simulink model "Figure8"  (R2021b)
settings: Solver=VariableStepAuto  StartTime=0.0  StopTime=10.0  RelTol=1e-3
undefined symbols (not defined in the file or in its folder): get, gray, res
libraries: myLib_CustomBoolean x15, dspobslib x1
settings Model: Creator=matt  LastModifiedBy=matt

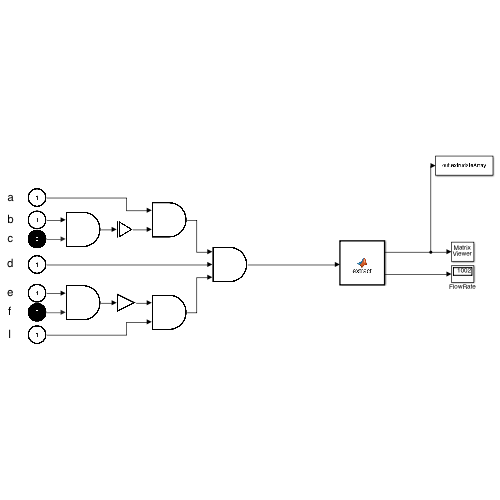
[thumbnail: Simulink's stored preview of the top-level diagram]
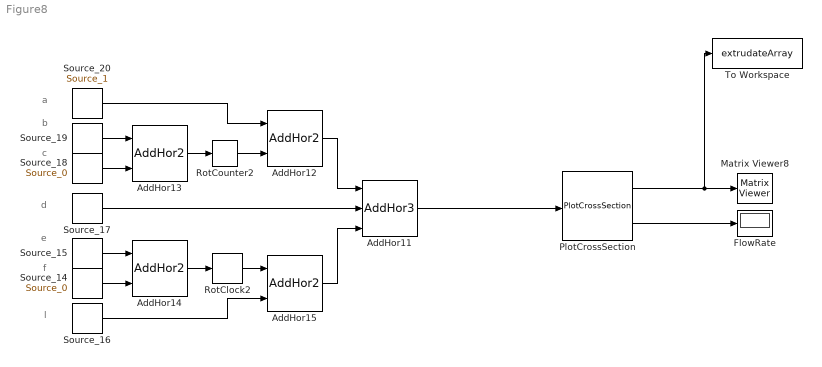
== system Figure8 ==
  note: l
  note: f
  note: d
  note: c
  note: e
  note: b
  note: a
  AddHor11 : myLib_CustomBoolean/AddHor3  SystemSampleTime=-1  VariantActivationTime=update diagram  Latency=0  AutoFrameSizeCalculation=off
      settings: SourceProductName=Boolean_Custom_Library
  AddHor{12..15} (4 alike) : myLib_CustomBoolean/AddHor2  SystemSampleTime=-1  VariantActivationTime=update diagram  Latency=0  AutoFrameSizeCalculation=off
      settings: SourceProductName=Boolean_Custom_Library
  FlowRate : Display
  Matrix Viewer8 : dspobslib/Matrix Viewer  ImageParams=off  CMapStr=gray(3)  AxisColorbar=on  AxisParams=off  AxisOrigin=Upper left corner  AxisTickMode=User-defined  XTickRange=[0 1]  YTickRange=[0 1]  XLabel=X-axis  YLabel=Y-axis  ZLabel=Z-axis  FigPos=get(0,'defaultfigureposition')  AxisZoom=off
      settings: SourceProductBaseCode=DS  YMin=0  YMax=1
  PlotCrossSection : myLib_CustomBoolean/PlotCrossSection  SystemSampleTime=-1  VariantActivationTime=update diagram  Latency=0  AutoFrameSizeCalculation=off
      settings: SourceProductName=Boolean_Custom_Library
  RotClock2 : myLib_CustomBoolean/RotClock  SystemSampleTime=-1  VariantActivationTime=update diagram  Latency=0  AutoFrameSizeCalculation=off
      settings: SourceProductName=Boolean_Custom_Library
  RotCounter2 : myLib_CustomBoolean/RotCounter  SystemSampleTime=-1  VariantActivationTime=update diagram  Latency=0  AutoFrameSizeCalculation=off
      settings: SourceProductName=Boolean_Custom_Library
  Source_14 : myLib_CustomBoolean/Source_0  Value=cat(3, 0.*ones(res,res), 150.*ones(res,res))  VectorParams1D=off  OutMin=[]  OutMax=[]  OutDataTypeStr=Inherit: Inherit from 'Constant value'  SampleTime=inf  FramePeriod=inf
      settings: SourceProductName=Boolean_Custom_Library
  Source_15 : myLib_CustomBoolean/Source_1  Value=cat(3, 1.*ones(res,res), 17*ones(res,res))  VectorParams1D=off  OutMin=[]  OutMax=[]  OutDataTypeStr=Inherit: Inherit from 'Constant value'  SampleTime=inf  FramePeriod=inf
      settings: SourceProductName=Boolean_Custom_Library
  Source_16 : myLib_CustomBoolean/Source_1  Value=cat(3, 1.*ones(res,res), 167*ones(res,res))  VectorParams1D=off  OutMin=[]  OutMax=[]  OutDataTypeStr=Inherit: Inherit from 'Constant value'  SampleTime=inf  FramePeriod=inf
      settings: SourceProductName=Boolean_Custom_Library
  Source_17 : myLib_CustomBoolean/Source_1  Value=cat(3, 1.*ones(res,res), 334*ones(res,res))  VectorParams1D=off  OutMin=[]  OutMax=[]  OutDataTypeStr=Inherit: Inherit from 'Constant value'  SampleTime=inf  FramePeriod=inf
      settings: SourceProductName=Boolean_Custom_Library
  Source_18 : myLib_CustomBoolean/Source_0  Value=cat(3, 0.*ones(res,res), 150.*ones(res,res))  VectorParams1D=off  OutMin=[]  OutMax=[]  OutDataTypeStr=Inherit: Inherit from 'Constant value'  SampleTime=inf  FramePeriod=inf
      settings: SourceProductName=Boolean_Custom_Library
  Source_19 : myLib_CustomBoolean/Source_1  Value=cat(3, 1.*ones(res,res), 17*ones(res,res))  VectorParams1D=off  OutMin=[]  OutMax=[]  OutDataTypeStr=Inherit: Inherit from 'Constant value'  SampleTime=inf  FramePeriod=inf
      settings: SourceProductName=Boolean_Custom_Library
  Source_20 : myLib_CustomBoolean/Source_1  Value=cat(3, 1.*ones(res,res), 167*ones(res,res))  VectorParams1D=off  OutMin=[]  OutMax=[]  OutDataTypeStr=Inherit: Inherit from 'Constant value'  SampleTime=inf  FramePeriod=inf
      settings: SourceProductName=Boolean_Custom_Library
  To Workspace : ToWorkspace  VariableName=extrudateArray  SampleTime=51
  wires:
  Source_17/1 -> AddHor11/2
  RotCounter2/1 -> AddHor12/2
  AddHor11/1 -> PlotCrossSection/1
  Source_16/1 -> AddHor15/2
  Source_20/1 -> AddHor12/1
  Source_14/1 -> AddHor14/2
  AddHor13/1 -> RotCounter2/1
  Source_15/1 -> AddHor14/1
  AddHor14/1 -> RotClock2/1
  AddHor12/1 -> AddHor11/1
  PlotCrossSection/2 -> FlowRate/1
  Source_19/1 -> AddHor13/1
  Source_18/1 -> AddHor13/2
  RotClock2/1 -> AddHor15/1
  AddHor15/1 -> AddHor11/3
  PlotCrossSection/1 -> To Workspace/1, Matrix Viewer8/1
